simulink model "ControleOrbital"  (R2023b)
settings: Solver=FixedStepAuto  StartTime=0.0  StopTime=tf  FixedStep=step_modelo  MaxStep=1  MinStep=0.1  RelTol=1e-12  AbsTol=1e-12
undefined symbols (not defined in the file or in its folder): man, OrbKd_x, OrbKd_y, OrbKd_z, OrbKi_x, OrbKi_y, OrbKi_z, OrbKp_x, OrbKp_y, OrbKp_z
settings Model: PacingRate=447  Creator=rodri  LastModifiedBy=rodri
settings SolverCC: NumberNewtonIterations=10

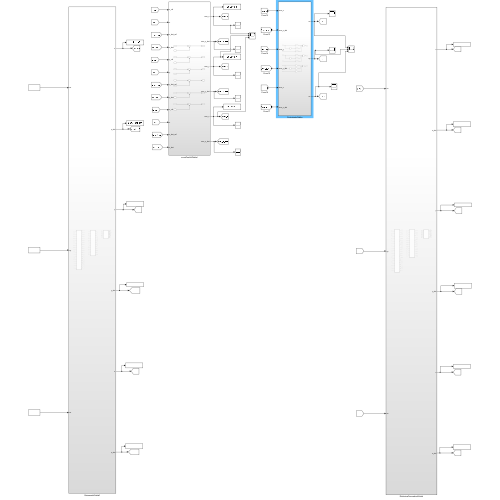
[thumbnail: Simulink's stored preview of the top-level diagram]
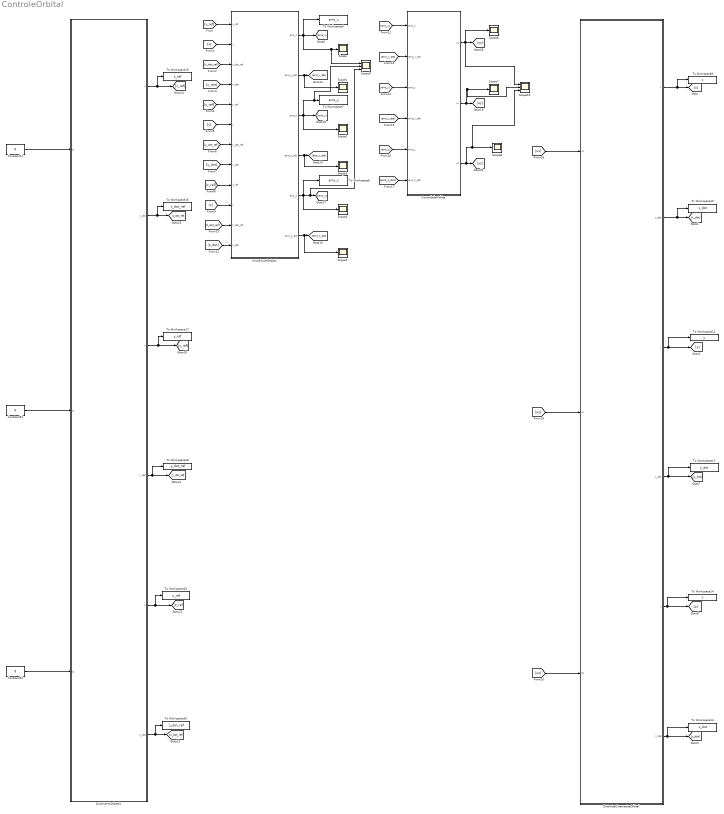
== system ControleOrbital ==
  Constant17 : Constant  Value=0
  Constant53 : Constant  Value=0
  Constant54 : Constant  Value=0
  ControladorOrbita : Subsystem
  DinâmicaCinematicaOrbital : Subsystem
  GuiamentoOrbital1 : Subsystem
  Scope{,1..8} (9 alike) : Scope
  Scope10 : Scope  NumInputPorts=3
  Scope9 : Scope  NumInputPorts=3
  To Workspace10 : ToWorkspace  VariableName=x_dot  SaveFormat=Timeseries  SampleTime=-1
  To Workspace11 : ToWorkspace  VariableName=y_dot  SaveFormat=Timeseries  SampleTime=-1
  To Workspace12 : ToWorkspace  VariableName=y  SaveFormat=Timeseries  SampleTime=-1
  To Workspace13 : ToWorkspace  VariableName=z_dot  SaveFormat=Timeseries  SampleTime=-1
  To Workspace14 : ToWorkspace  VariableName=z  SaveFormat=Timeseries  SampleTime=-1
  To Workspace15 : ToWorkspace  VariableName=x_ref  SaveFormat=Timeseries  SampleTime=-1
  To Workspace16 : ToWorkspace  VariableName=x_dot_ref  SaveFormat=Timeseries  SampleTime=-1
  To Workspace17 : ToWorkspace  VariableName=y_ref  SaveFormat=Timeseries  SampleTime=-1
  To Workspace18 : ToWorkspace  VariableName=y_dot_ref  SaveFormat=Timeseries  SampleTime=-1
  To Workspace19 : ToWorkspace  VariableName=z_ref  SaveFormat=Timeseries  SampleTime=-1
  To Workspace20 : ToWorkspace  VariableName=z_dot_ref  SaveFormat=Timeseries  SampleTime=-1
  To Workspace6 : ToWorkspace  VariableName=erro_x  SaveFormat=Timeseries  SampleTime=-1
  To Workspace7 : ToWorkspace  VariableName=erro_y  SaveFormat=Timeseries  SampleTime=-1
  To Workspace8 : ToWorkspace  VariableName=erro_z  SaveFormat=Timeseries  SampleTime=-1
  To Workspace9 : ToWorkspace  VariableName=x  SaveFormat=Timeseries  SampleTime=-1
  errosPosVelOrbital : Subsystem
  wires:
  [erro_x] -> ControladorOrbita/1(erro_x)
  ControladorOrbita/1(ux) -> Scope10/1, Scope6/1, [ux]
  [erro_y_dot] -> ControladorOrbita/4(erro_y_dot)
  [erro_x_dot] -> ControladorOrbita/2(erro_x_dot)
  ControladorOrbita/2(uy) -> Scope10/2, Scope7/1, [uy]
  [erro_y] -> ControladorOrbita/3(erro_y)
  [erro_z_dot] -> ControladorOrbita/6(erro_z_dot)
  [erro_z] -> ControladorOrbita/5(erro_z)
  ControladorOrbita/3(uz) -> Scope10/3, Scope8/1, [uz]
  [x_ref] -> errosPosVelOrbital/1(x_ref)
  [x] -> errosPosVelOrbital/2(x)
  [x_dot_ref] -> errosPosVelOrbital/3(x_dot_ref)
  [x_dot] -> errosPosVelOrbital/4(x_dot)
  [y_ref] -> errosPosVelOrbital/5(y_ref)
  [y] -> errosPosVelOrbital/6(y)
  [y_dot_ref] -> errosPosVelOrbital/7(y_dot_ref)
  [y_dot] -> errosPosVelOrbital/8(y_dot)
  [z] -> errosPosVelOrbital/10(z)
  [z_dot_ref] -> errosPosVelOrbital/11(z_dot_ref)
  [z_dot] -> errosPosVelOrbital/12(z_dot)
  [z_ref] -> errosPosVelOrbital/9(z_ref)
  errosPosVelOrbital/1(erro_x) -> Scope/1, Scope9/1, [erro_x], To Workspace6/1
  errosPosVelOrbital/2(erro_x_dot) -> Scope1/1, [erro_x_dot]
  errosPosVelOrbital/4(erro_y_dot) -> Scope3/1, [erro_y_dot]
  errosPosVelOrbital/3(erro_y) -> Scope2/1, Scope9/2, To Workspace7/1, [erro_y]
  errosPosVelOrbital/6(erro_z_dot) -> Scope5/1, [erro_z_dot]
  errosPosVelOrbital/5(erro_z) -> Scope4/1, To Workspace8/1, [erro_z], Scope9/3
  GuiamentoOrbital1/1(x) -> To Workspace15/1, [x_ref]
  GuiamentoOrbital1/5(z) -> To Workspace19/1, [z_ref]
  Constant54/1 -> GuiamentoOrbital1/3(uz)
  Constant17/1 -> GuiamentoOrbital1/1(ux)
  GuiamentoOrbital1/4(y_dot) -> To Workspace18/1, [y_dot_ref]
  Constant53/1 -> GuiamentoOrbital1/2(uy)
  GuiamentoOrbital1/3(y) -> [y_ref], To Workspace17/1
  GuiamentoOrbital1/2(x_dot) -> [x_dot_ref], To Workspace16/1
  GuiamentoOrbital1/6(z_dot) -> To Workspace20/1, [z_dot_ref]
  DinâmicaCinematicaOrbital/3(y) -> [y], To Workspace12/1
  DinâmicaCinematicaOrbital/1(x) -> To Workspace9/1, [x]
  [uy] -> DinâmicaCinematicaOrbital/2(uy)
  [ux] -> DinâmicaCinematicaOrbital/1(ux)
  [uz] -> DinâmicaCinematicaOrbital/3(uz)
  DinâmicaCinematicaOrbital/4(y_dot) -> To Workspace11/1, [y_dot]
  DinâmicaCinematicaOrbital/6(z_dot) -> [z_dot], To Workspace13/1
  DinâmicaCinematicaOrbital/5(z) -> To Workspace14/1, [z]
  DinâmicaCinematicaOrbital/2(x_dot) -> To Workspace10/1, [x_dot]

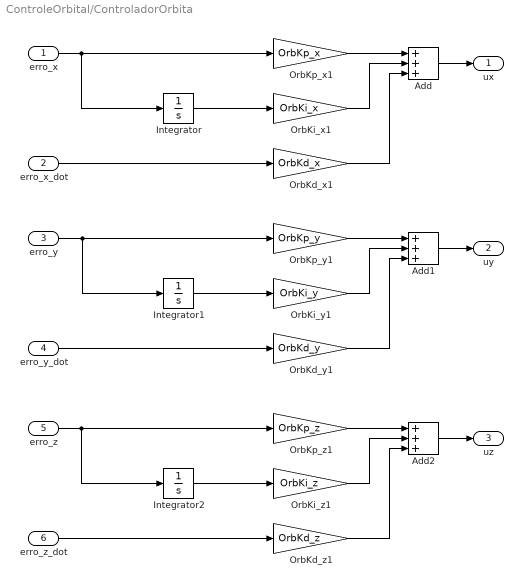
== system ControleOrbital/ControladorOrbita ==
  erro_x : Inport
  erro_x_dot : Inport  Port=2
  erro_y : Inport  Port=3
  erro_y_dot : Inport  Port=4
  erro_z : Inport  Port=5
  erro_z_dot : Inport  Port=6
  Add : Sum  Inputs=+++
  Add1 : Sum  Inputs=+++
  Add2 : Sum  Inputs=+++
  Integrator : Integrator
  Integrator1 : Integrator
  Integrator2 : Integrator
  OrbKd_x1 : Gain  Gain=OrbKd_x
  OrbKd_y1 : Gain  Gain=OrbKd_y
  OrbKd_z1 : Gain  Gain=OrbKd_z
  OrbKi_x1 : Gain  Gain=OrbKi_x
  OrbKi_y1 : Gain  Gain=OrbKi_y
  OrbKi_z1 : Gain  Gain=OrbKi_z
  OrbKp_x1 : Gain  Gain=OrbKp_x
  OrbKp_y1 : Gain  Gain=OrbKp_y
  OrbKp_z1 : Gain  Gain=OrbKp_z
  ux : Outport
  uy : Outport  Port=2
  uz : Outport  Port=3
  wires:
  OrbKd_x1/1 -> Add/3
  OrbKi_x1/1 -> Add/2
  OrbKp_x1/1 -> Add/1
  Add/1 -> ux/1
  OrbKd_y1/1 -> Add1/3
  OrbKp_y1/1 -> Add1/1
  Add1/1 -> uy/1
  OrbKi_y1/1 -> Add1/2
  Add2/1 -> uz/1
  OrbKi_z1/1 -> Add2/2
  OrbKd_z1/1 -> Add2/3
  OrbKp_z1/1 -> Add2/1
  erro_x/1 -> OrbKp_x1/1, Integrator/1
  Integrator/1 -> OrbKi_x1/1
  erro_x_dot/1 -> OrbKd_x1/1
  erro_y/1 -> OrbKp_y1/1, Integrator1/1
  Integrator1/1 -> OrbKi_y1/1
  erro_y_dot/1 -> OrbKd_y1/1
  erro_z/1 -> OrbKp_z1/1, Integrator2/1
  Integrator2/1 -> OrbKi_z1/1
  erro_z_dot/1 -> OrbKd_z1/1

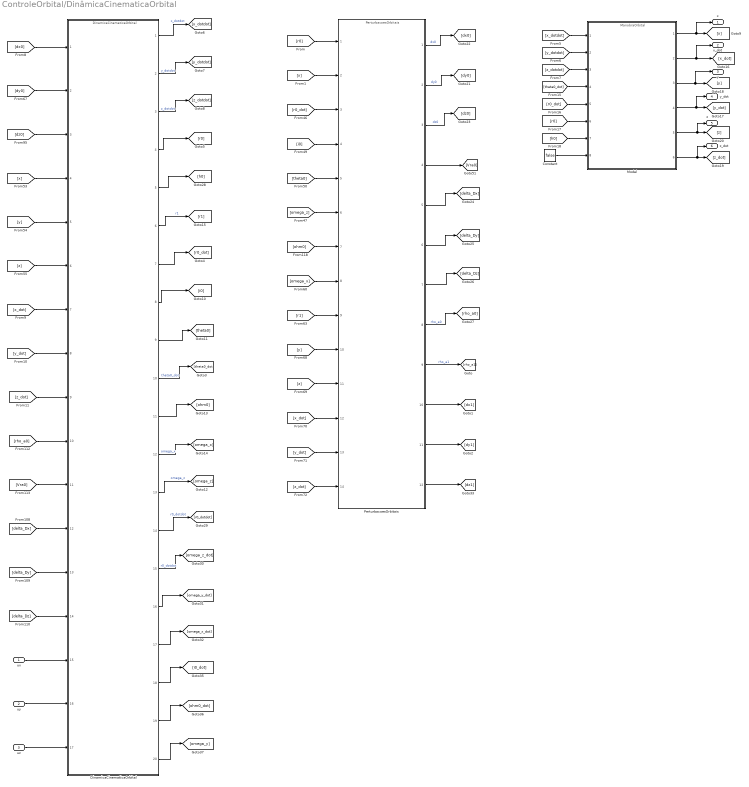
== system ControleOrbital/DinâmicaCinematicaOrbital ==
  ux : Inport  OutDataTypeStr=double  PortDimensions=1
  uy : Inport  Port=2  OutDataTypeStr=double  PortDimensions=1
  uz : Inport  Port=3  OutDataTypeStr=double  PortDimensions=1
  Constant : Constant  Value=false
  DinamicaCinematicaOrbital : ModelReference  ModelNameDialog=DinamicaCinematicaOrbital  ModelReferenceVersion=4.0
  Model : ModelReference  ModelNameDialog=ManobraOrbital.slx  ModelReferenceVersion=4.2
  PerturbacoesOrbitais : ModelReference  ModelNameDialog=PerturbacoesOrbitais  ModelReferenceVersion=4.0
  x : Outport  OutDataTypeStr=double  PortDimensions=1  SampleTime=0
  x_dot : Outport  Port=2  OutDataTypeStr=double  PortDimensions=1  SampleTime=0
  y : Outport  Port=3  OutDataTypeStr=double  PortDimensions=1  SampleTime=0
  y_dot : Outport  Port=4  OutDataTypeStr=double  PortDimensions=1  SampleTime=0
  z : Outport  Port=5  OutDataTypeStr=double  PortDimensions=1  SampleTime=0
  z_dot : Outport  Port=6  OutDataTypeStr=double  PortDimensions=1  SampleTime=0
  wires:
  [delta_Dz] -> DinamicaCinematicaOrbital/14
  DinamicaCinematicaOrbital/16 -> [omega_y_dot]
  [r0] -> Model/6
  [theta0_dot] -> Model/4
  [h0] -> Model/7
  [y] -> PerturbacoesOrbitais/10
  [omega_x] -> PerturbacoesOrbitais/8
  PerturbacoesOrbitais/3 -> [dz0]  "dz0"
  [z_dot] -> DinamicaCinematicaOrbital/9
  DinamicaCinematicaOrbital/19 -> [ohm0_dot]
  [x_dot] -> PerturbacoesOrbitais/12
  [y_dotdot] -> Model/2
  DinamicaCinematicaOrbital/14 -> [r0_dotdot]  "r0_dotdot"
  [z_dot] -> PerturbacoesOrbitais/14
  [x_dotdot] -> Model/1
  [z] -> PerturbacoesOrbitais/11
  [delta_Dx] -> DinamicaCinematicaOrbital/12
  PerturbacoesOrbitais/1 -> [dx0]  "dx0"
  [y_dot] -> PerturbacoesOrbitais/13
  DinamicaCinematicaOrbital/3 -> [z_dotdot]  "z_dotdot"
  DinamicaCinematicaOrbital/13 -> [omega_z]  "omega_z"
  Model/2 -> x_dot/1, [x_dot]
  uz/1 -> DinamicaCinematicaOrbital/17
  DinamicaCinematicaOrbital/4 -> [r0]
  [omega_z] -> PerturbacoesOrbitais/6
  [r1] -> PerturbacoesOrbitais/9
  [delta_Dy] -> DinamicaCinematicaOrbital/13
  [ohm0] -> PerturbacoesOrbitais/7
  [r0] -> PerturbacoesOrbitais/1
  [dx0] -> DinamicaCinematicaOrbital/1
  uy/1 -> DinamicaCinematicaOrbital/16
  Model/3 -> y/1, [y]
  [i0] -> PerturbacoesOrbitais/4
  [x] -> PerturbacoesOrbitais/2
  [r0_dot] -> PerturbacoesOrbitais/3
  [dy0] -> DinamicaCinematicaOrbital/2
  [Vra0] -> DinamicaCinematicaOrbital/11
  Model/5 -> [z], z/1
  DinamicaCinematicaOrbital/5 -> [h0]
  [y] -> DinamicaCinematicaOrbital/5
  [z] -> DinamicaCinematicaOrbital/6
  ux/1 -> DinamicaCinematicaOrbital/15
  Model/1 -> x/1, [x]
  DinamicaCinematicaOrbital/15 -> [omega_z_dot]  "r0_dotdot"
  [dz0] -> DinamicaCinematicaOrbital/3
  DinamicaCinematicaOrbital/17 -> [omega_x_dot]
  Constant/1 -> Model/8
  DinamicaCinematicaOrbital/11 -> [ohm0]
  [rho_a0] -> DinamicaCinematicaOrbital/10
  DinamicaCinematicaOrbital/7 -> [r0_dot]
  DinamicaCinematicaOrbital/18 -> [i0_dot]
  DinamicaCinematicaOrbital/20 -> [omega_y]
  DinamicaCinematicaOrbital/2 -> [y_dotdot]  "y_dotdot"
  [r0_dot] -> Model/5
  Model/6 -> z_dot/1, [z_dot]
  DinamicaCinematicaOrbital/10 -> [theta0_dot]  "theta0_dot"
  [x] -> DinamicaCinematicaOrbital/4
  DinamicaCinematicaOrbital/12 -> [omega_x]  "omega_x"
  PerturbacoesOrbitais/4 -> [Vra0]
  [theta0] -> PerturbacoesOrbitais/5
  DinamicaCinematicaOrbital/8 -> [i0]
  [z_dotdot] -> Model/3
  DinamicaCinematicaOrbital/6 -> [r1]  "r1"
  PerturbacoesOrbitais/8 -> [rho_a0]  "rho_a0"
  [y_dot] -> DinamicaCinematicaOrbital/8
  PerturbacoesOrbitais/5 -> [delta_Dx]
  Model/4 -> y_dot/1, [y_dot]
  PerturbacoesOrbitais/2 -> [dy0]  "dy0"
  PerturbacoesOrbitais/6 -> [delta_Dy]
  DinamicaCinematicaOrbital/1 -> [x_dotdot]  "x_dotdot"
  [x_dot] -> DinamicaCinematicaOrbital/7
  PerturbacoesOrbitais/7 -> [delta_Dz]
  DinamicaCinematicaOrbital/9 -> [theta0]
  PerturbacoesOrbitais/9 -> [rho_a1]  "rho_a1"
  PerturbacoesOrbitais/10 -> [dx1]
  PerturbacoesOrbitais/11 -> [dy1]
  PerturbacoesOrbitais/12 -> [dz1]

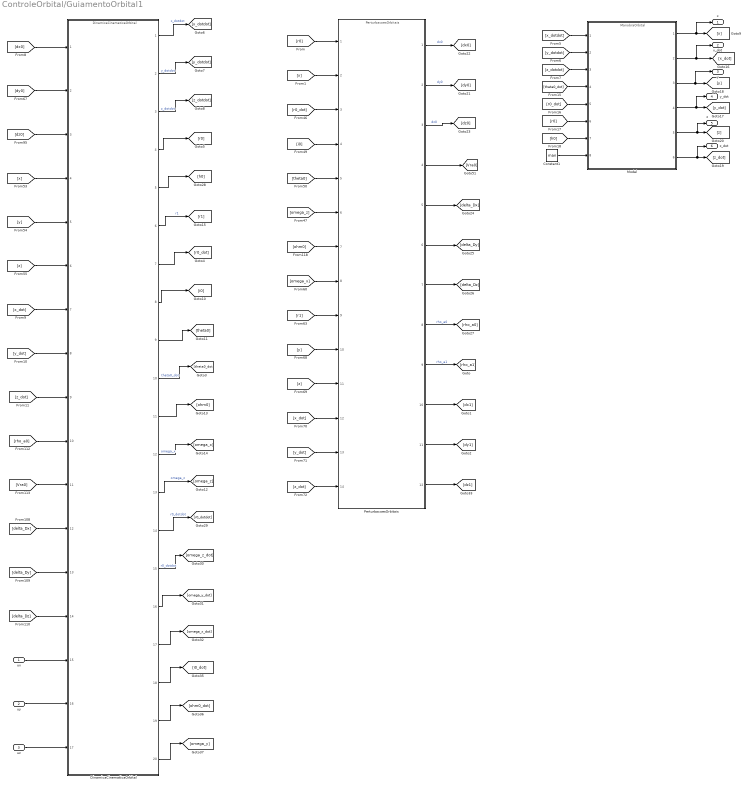
== system ControleOrbital/GuiamentoOrbital1 ==
  ux : Inport  OutDataTypeStr=double  PortDimensions=1
  uy : Inport  Port=2  OutDataTypeStr=double  PortDimensions=1
  uz : Inport  Port=3  OutDataTypeStr=double  PortDimensions=1
  Constant1 : Constant  Value=man
  DinamicaCinematicaOrbital : ModelReference  ModelNameDialog=DinamicaCinematicaOrbital  ModelReferenceVersion=4.0
  Model : ModelReference  ModelNameDialog=ManobraOrbital.slx  ModelReferenceVersion=4.2
  PerturbacoesOrbitais : ModelReference  ModelNameDialog=PerturbacoesOrbitais  ModelReferenceVersion=4.0
  x : Outport  OutDataTypeStr=double  PortDimensions=1  SampleTime=0
  x_dot : Outport  Port=2  OutDataTypeStr=double  PortDimensions=1  SampleTime=0
  y : Outport  Port=3  OutDataTypeStr=double  PortDimensions=1  SampleTime=0
  y_dot : Outport  Port=4  OutDataTypeStr=double  PortDimensions=1  SampleTime=0
  z : Outport  Port=5  OutDataTypeStr=double  PortDimensions=1  SampleTime=0
  z_dot : Outport  Port=6  OutDataTypeStr=double  PortDimensions=1  SampleTime=0
  wires:
  [delta_Dz] -> DinamicaCinematicaOrbital/14
  DinamicaCinematicaOrbital/16 -> [omega_y_dot]
  [r0] -> Model/6
  [theta0_dot] -> Model/4
  [h0] -> Model/7
  [y] -> PerturbacoesOrbitais/10
  [omega_x] -> PerturbacoesOrbitais/8
  PerturbacoesOrbitais/3 -> [dz0]  "dz0"
  [z_dot] -> DinamicaCinematicaOrbital/9
  DinamicaCinematicaOrbital/19 -> [ohm0_dot]
  [x_dot] -> PerturbacoesOrbitais/12
  [y_dotdot] -> Model/2
  DinamicaCinematicaOrbital/14 -> [r0_dotdot]  "r0_dotdot"
  [z_dot] -> PerturbacoesOrbitais/14
  [x_dotdot] -> Model/1
  [z] -> PerturbacoesOrbitais/11
  [delta_Dx] -> DinamicaCinematicaOrbital/12
  PerturbacoesOrbitais/1 -> [dx0]  "dx0"
  [y_dot] -> PerturbacoesOrbitais/13
  DinamicaCinematicaOrbital/3 -> [z_dotdot]  "z_dotdot"
  DinamicaCinematicaOrbital/13 -> [omega_z]  "omega_z"
  Model/2 -> x_dot/1, [x_dot]
  uz/1 -> DinamicaCinematicaOrbital/17
  DinamicaCinematicaOrbital/4 -> [r0]
  [omega_z] -> PerturbacoesOrbitais/6
  [r1] -> PerturbacoesOrbitais/9
  [delta_Dy] -> DinamicaCinematicaOrbital/13
  [ohm0] -> PerturbacoesOrbitais/7
  [r0] -> PerturbacoesOrbitais/1
  [dx0] -> DinamicaCinematicaOrbital/1
  uy/1 -> DinamicaCinematicaOrbital/16
  Model/3 -> y/1, [y]
  [i0] -> PerturbacoesOrbitais/4
  [x] -> PerturbacoesOrbitais/2
  [r0_dot] -> PerturbacoesOrbitais/3
  [dy0] -> DinamicaCinematicaOrbital/2
  [Vra0] -> DinamicaCinematicaOrbital/11
  Model/5 -> [z], z/1
  DinamicaCinematicaOrbital/5 -> [h0]
  [y] -> DinamicaCinematicaOrbital/5
  [z] -> DinamicaCinematicaOrbital/6
  ux/1 -> DinamicaCinematicaOrbital/15
  Model/1 -> x/1, [x]
  DinamicaCinematicaOrbital/15 -> [omega_z_dot]  "r0_dotdot"
  [dz0] -> DinamicaCinematicaOrbital/3
  DinamicaCinematicaOrbital/17 -> [omega_x_dot]
  Constant1/1 -> Model/8
  DinamicaCinematicaOrbital/11 -> [ohm0]
  [rho_a0] -> DinamicaCinematicaOrbital/10
  DinamicaCinematicaOrbital/7 -> [r0_dot]
  DinamicaCinematicaOrbital/18 -> [i0_dot]
  DinamicaCinematicaOrbital/20 -> [omega_y]
  DinamicaCinematicaOrbital/2 -> [y_dotdot]  "y_dotdot"
  [r0_dot] -> Model/5
  Model/6 -> z_dot/1, [z_dot]
  DinamicaCinematicaOrbital/10 -> [theta0_dot]  "theta0_dot"
  [x] -> DinamicaCinematicaOrbital/4
  DinamicaCinematicaOrbital/12 -> [omega_x]  "omega_x"
  PerturbacoesOrbitais/4 -> [Vra0]
  [theta0] -> PerturbacoesOrbitais/5
  DinamicaCinematicaOrbital/8 -> [i0]
  [z_dotdot] -> Model/3
  DinamicaCinematicaOrbital/6 -> [r1]  "r1"
  PerturbacoesOrbitais/8 -> [rho_a0]  "rho_a0"
  [y_dot] -> DinamicaCinematicaOrbital/8
  PerturbacoesOrbitais/5 -> [delta_Dx]
  Model/4 -> y_dot/1, [y_dot]
  PerturbacoesOrbitais/2 -> [dy0]  "dy0"
  PerturbacoesOrbitais/6 -> [delta_Dy]
  DinamicaCinematicaOrbital/1 -> [x_dotdot]  "x_dotdot"
  [x_dot] -> DinamicaCinematicaOrbital/7
  PerturbacoesOrbitais/7 -> [delta_Dz]
  DinamicaCinematicaOrbital/9 -> [theta0]
  PerturbacoesOrbitais/9 -> [rho_a1]  "rho_a1"
  PerturbacoesOrbitais/10 -> [dx1]
  PerturbacoesOrbitais/11 -> [dy1]
  PerturbacoesOrbitais/12 -> [dz1]

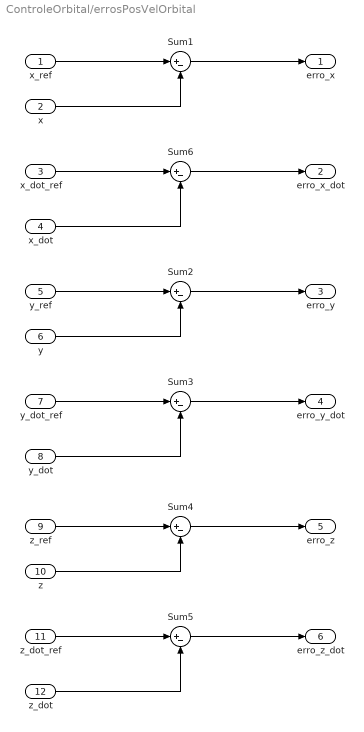
== system ControleOrbital/errosPosVelOrbital ==
  x_ref : Inport
  x : Inport  Port=2
  x_dot_ref : Inport  Port=3
  x_dot : Inport  Port=4
  y_ref : Inport  Port=5
  y : Inport  Port=6
  y_dot_ref : Inport  Port=7
  y_dot : Inport  Port=8
  z_ref : Inport  Port=9
  z : Inport  Port=10
  z_dot_ref : Inport  Port=11
  z_dot : Inport  Port=12
  Sum{1..6} (6 alike) : Sum  Inputs=|+-
  erro_x : Outport
  erro_x_dot : Outport  Port=2
  erro_y : Outport  Port=3
  erro_y_dot : Outport  Port=4
  erro_z : Outport  Port=5
  erro_z_dot : Outport  Port=6
  wires:
  x/1 -> Sum1/2
  x_dot/1 -> Sum6/2
  x_dot_ref/1 -> Sum6/1
  x_ref/1 -> Sum1/1
  Sum6/1 -> erro_x_dot/1
  Sum1/1 -> erro_x/1
  Sum3/1 -> erro_y_dot/1
  Sum2/1 -> erro_y/1
  y/1 -> Sum2/2
  y_dot/1 -> Sum3/2
  y_ref/1 -> Sum2/1
  y_dot_ref/1 -> Sum3/1
  Sum5/1 -> erro_z_dot/1
  Sum4/1 -> erro_z/1
  z_dot/1 -> Sum5/2
  z_dot_ref/1 -> Sum5/1
  z/1 -> Sum4/2
  z_ref/1 -> Sum4/1
